simulink model "MpcRefMdl"  (R2019a)
settings: Solver=FixedStepAuto  StartTime=0.0  StopTime=100  FixedStep=0.005  MaxStep=1e-2  MinStep=1e-3  RelTol=5e-3
values from neighbouring files (symbols this model uses):
  wheelbase = 0.3    [createCostmap.m]
libraries: mpcadaslib x1, simulink x1, simulink_extras x1
settings Model: Creator=The MathWorks, Inc.  LastModifiedBy=mingz
settings SolverCC: ZeroCrossAlgorithm=Adaptive  DecoupledContinuousIntegration=on  MinimalZcImpactIntegration=on
settings DataIOCC: SaveOutput=off  SignalLogging=off  DSMLogging=off  SaveTime=off  ReturnWorkspaceOutputs=off
settings DebuggingCC: PregeneratedLibrarySubsystemCodeDiagnostic=none  ArithmeticOperatorsInVariantConditions=warning
settings SFSimCC: SimUseLocalCustomCode=off
settings RTWCC: RTWUseLocalCustomCode=off

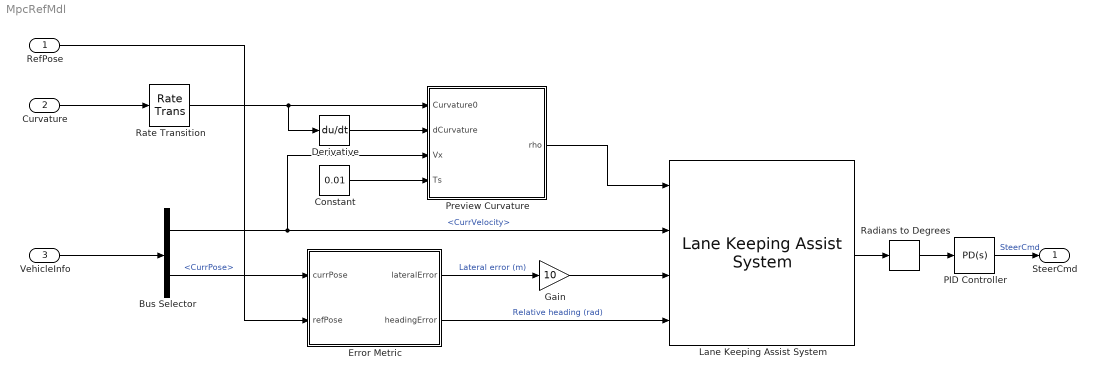
== system MpcRefMdl ==
  RefPose : Inport
  Curvature : Inport  Port=2
  VehicleInfo : Inport  Port=3  OutDataTypeStr=Bus: vehicleInfoBus
  Bus Selector : BusSelector  OutputSignals=CurrVelocity,CurrPose
  Constant : Constant  Value=0.01
  Derivative : Derivative
  Error Metric : MATLAB Function  TreatAsAtomicUnit=on  mask{wheelbase=wheelbase}
      mask prompts: wheelbase "Wheelbase of vehicle"
  Gain : Gain  Gain=10
  Lane Keeping Assist System : mpcadaslib/Lane Keeping Assist System  ModelType=Use vehicle parameters  VehicleMass=1.2  VehicleYawInertia=0.004  LengthToFront=0.10  LengthToRear=0.05  FrontTireStiffness=19000  RearTireStiffness=35000  EgoModelMatrixA=[-4.4021 ,-12.4603;1.3913,-5.1868]  EgoModelMatrixB=[24.1270;15.8609]  EgoModelMatrixC=[1,0;0,1]  InitialLongVel=1  TransportLag=0  MinSteering=-0.61  umin_ext=off  MaxSteering=0.61  umax_ext=off  Ts=0.01  PredictionHorizon=10  ControllerBehavior=0.3  suboptimal=off  maxiter=10  datatypeopt=double  optmode=off  trackmode=off
      settings: SourceProductName=MATLAB Runtime - Model Predictive Control Toolbox Addin  SourceProductBaseCode=Missing
  PID Controller : simulink/Continuous/PID Controller  Controller=PD  Form=Parallel  TimeDomain=Continuous-time  SampleTime=-1  IntegratorMethod=Forward Euler  FilterMethod=Forward Euler  ControllerParametersSource=internal  P=1  I=1  D=0.01  UseFilter=on  N=100  TunerSelectOption=Transfer Function Based (PID Tuner App)  InitialConditionSource=internal  InitialConditionForIntegrator=0  InitialConditionForFilter=0  DifferentiatorICPrevScaledInput=0  ExternalReset=none  TrackingMode=off  Kt=1  LimitOutput=off  UpperSaturationLimit=inf  LowerSaturationLimit=-inf  LinearizeAsGain=on  AntiWindupMode=none  Kb=1  POutMin=[]  POutMax=[]  IOutMin=[]  IOutMax=[]  DOutMin=[]  DOutMax=[]  NOutMin=[]  NOutMax=[]  SumOutMin=[]  SumOutMax=[]  SaturationOutMin=[]  SaturationOutMax=[]  PParamMin=[]  PParamMax=[]  IParamMin=[]  IParamMax=[]  DParamMin=[]  DParamMax=[]  NParamMin=[]  NParamMax=[]  KbParamMin=[]  KbParamMax=[]  KtParamMin=[]  KtParamMax=[]  KbOutMin=[]  KbOutMax=[]  KtOutMin=[]  KtOutMax=[]  IntegratorOutMin=[]  IntegratorOutMax=[]  FilterOutMin=[]  FilterOutMax=[]  SumI1OutMin=[]  SumI1OutMax=[]  SumI2OutMin=[]  SumI2OutMax=[]  SumI3OutMin=[]  SumI3OutMax=[]  SumI4OutMin=[]  SumI4OutMax=[]  SumDOutMin=[]  SumDOutMax=[]  DifferentiatorOutMin=[]  DifferentiatorOutMax=[]  FilterDiffOutCoefMin=[]  FilterDiffOutCoefMax=[]  ReciprocalOutMin=[]  ReciprocalOutMax=[]  SumDenOutMin=[]  SumDenOutMax=[]  SumNumOutMin=[]  SumNumOutMax=[]  DivideOutMin=[]  DivideOutMax=[]  IntegratorContinuousStateAttributes=''  IntegratorStateMustResolveToSignalObject=off  IntegratorRTWStateStorageClass=Auto  FilterContinuousStateAttributes=''  FilterStateMustResolveToSignalObject=off  FilterRTWStateStorageClass=Auto  ParallelPVariant=InternalParameters  IdealPVariant=Disabled  IVariant=Disabled  DVariant=InternalParameters  IntegratorVariant=Disabled  SatVariant=Disabled  AWVariant=Disabled  PCopyVariant=Disabled  TRVariant=Disabled  FdbkBlocksVariant=Forward  IdealPFdbkVariant=Disabled  SatFdbkVariant=Disabled  DerivativeFilterVariant=ContFilter  NVariant=InternalParameters  NCopyVariant=Disabled  FilterICVariant=InternalICsFilter  IntegratorICVariant=Disabled  ExternalResetVariant=Disabled  TRSumVariant=Passthrough  SumFdbkVariant=Disabled  SumVariant=Sum_PD
  Preview Curvature : MATLAB Function  TreatAsAtomicUnit=on
  Radians to Degrees : simulink_extras/Transformations/Radians to Degrees
  Rate Transition : RateTransition  OutPortSampleTime=0.01
  SteerCmd : Outport
  wires:
  Radians to Degrees/1 -> PID Controller/1
  VehicleInfo/1 -> Bus Selector/1
  Lane Keeping Assist System/1 -> Radians to Degrees/1
  Error Metric/1(lateralError) -> Gain/1  "Lateral error (m)"
  Error Metric/2(headingError) -> Lane Keeping Assist System/4  "Relative heading (rad)"
  Derivative/1 -> Preview Curvature/2(dCurvature)
  Bus Selector/1 -> Lane Keeping Assist System/2, Preview Curvature/3(Vx)  "<CurrVelocity>"
  Rate Transition/1 -> Derivative/1, Preview Curvature/1(Curvature0)
  Constant/1 -> Preview Curvature/4(Ts)
  Curvature/1 -> Rate Transition/1
  Bus Selector/2 -> Error Metric/1(currPose)  "<CurrPose>"
  Gain/1 -> Lane Keeping Assist System/3
  Preview Curvature/1(rho) -> Lane Keeping Assist System/1
  RefPose/1 -> Error Metric/2(refPose)
  PID Controller/1 -> SteerCmd/1  "SteerCmd"

== matlab function MpcRefMdl/Error Metric ==
  data: currPose input size=[1 3]; refPose input size=[1 3]; lateralError output; wheelbase parameter; headingError output
function [lateralError, headingError] = fcn(currPose, refPose, wheelbase)

%   Copyright 2018 The MathWorks, Inc.

currPose(:,3) = deg2rad(currPose(:,3));
refPose(:,3)  = deg2rad(refPose(:,3));

%Convert current pose to front wheel coordinate
currPoseF = driving.internal.control.rearPoseToFrontPose(currPose, wheelbase);

lateralError = norm(currPoseF(1:2) - refPose(1:2)) * ...
    sign( - sin(refPose(:,3)) * (currPoseF(1) - refPose(1)) ...
    + cos(refPose(:,3)) * (currPoseF(2) - refPose(2)));

d1 = rad2deg(currPose(:, 3) - refPose(:,3));
d2 = 360 - abs(d1);
if (d1>0)
    d2 = 0.0-d2;
end
if (abs(d1) < abs(d2))
    headingError = deg2rad(d1);
else
    headingError = deg2rad(d2);
end

== matlab function MpcRefMdl/Preview Curvature ==
  data: rho output size=11; Curvature0 input; dCurvature input; Vx input; Ts input
function rho = predictCurvature(Curvature0,dCurvature,Vx, Ts)
% Curvature0 = initial curvature per unit length                  [1/m]
% dCurvature = (constant) derivative of curvature per unit length [1/m^2]
% CurvatureLength = length for which the clothoid model is valid [m]
% Vx = speed of vehicle

% We want to export a set of curvatures at a uniform sample time ahead.
% t is this vector which goes up to 1 second in the future or having
% enough time to reach the known length in curvature (whichever is smaller)

% To enable truncation by curvelength, mark output "rho" as varsize
%t = 0:Ts:min(1,CurvatureLength/Vx);

t = zeros(11,1);
for i=1:numel(t)
    t(i) = (i-1).*Ts;
end

% We compute the curvature vector rho(t) using the specified clothoid model
rho = Curvature0 + dCurvature*Vx*t;
